simulink model "Force_control"  (R2020a)
settings: Solver=VariableStepAuto  StartTime=0.0  StopTime=10.0  RelTol=1e-3
values from neighbouring files (symbols this model uses):
  K = [C11 C12 C13 0 0 0; C12 C11 C13 0 0 0; C13 C13 C33 0 0 0; 0 0 0 C44 0 0; 0 0 0 0 C44 0; 0 0 0 0 0 C66]    [JoinScript.m]    (also in alldata.mat = [20.1 11.1 12 0 0 0 11.1 20.1 12 0 0 0 ... (36 elements, 6x6; aux_y2.m = Abb.fkine(q))
  Kd = 25*diag([1 1 1 1 1 1])    [JoinScript.m]    (also in alldata.mat = [150 0 0 0 0 0 0 150 0 0 0 0 ... (36 elements, 6x6)]; aux_y.m = 3e2*diag([1 1 1 1 1 1]); aux_y2.m = 3e2*diag([1 1 1 1 1 1]))
  Kp = 100*diag([0.01 1 1 1 1 1])    [JoinScript.m]    (also in alldata.mat = [200 0 0 0 0 0 0 200 0 0 0 0 ... (36 elements, 6x6)]; aux_y.m = 1e3*diag([1 1 1 1 1 1]); aux_y2.m = 1e3*diag([1 1 1 1 1 1]))
  x0 = dir_kin(qf)    [JoinScript.m]    (also in alldata.mat = [-5.32301496588e-18 0.480120382501 0.16494818601 1.570796326)
settings Model: Creator=doble  LastModifiedBy=doble

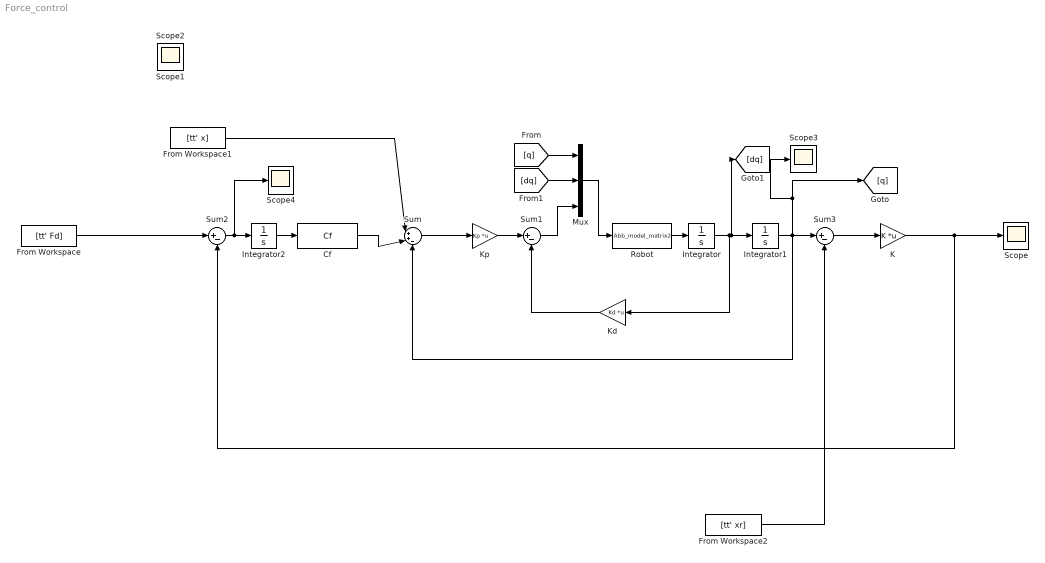
== system Force_control ==
  Cf : MATLABFcn  MATLABFcn=Cf  OutputDimensions=6*1
  From Workspace : FromWorkspace  VariableName=[tt' Fd]
  From Workspace1 : FromWorkspace  VariableName=[tt' x]
  From Workspace2 : FromWorkspace  VariableName=[tt' xr]
  Integrator : Integrator
  Integrator1 : Integrator  InitialCondition=x0
  Integrator2 : Integrator
  K : Gain  Gain=K  Multiplication=Matrix(K*u)
  Kd : Gain  Gain=Kd  Multiplication=Matrix(K*u)
  Kp : Gain  Gain=Kp  Multiplication=Matrix(K*u)
  Mux : Mux  Inputs=3
  Robot : MATLABFcn  MATLABFcn=Abb_model_matrix2  OutputDimensions=6*1
  Scope{,1..4} (5 alike) : Scope
  Sum : Sum  Inputs=|++-
  Sum1 : Sum  Inputs=|+-
  Sum2 : Sum  Inputs=|+-
  Sum3 : Sum  Inputs=|+-
  wires:
  From Workspace1/1 -> Sum/1
  Cf/1 -> Sum/2
  Sum/1 -> Kp/1
  Sum3/1 -> K/1
  Kp/1 -> Sum1/1
  Integrator/1 -> Kd/1, [dq], Integrator1/1
  Integrator1/1 -> [q], Scope3/1, Sum/3, Sum3/1
  Kd/1 -> Sum1/2
  K/1 -> Sum2/2, Scope/1
  From Workspace2/1 -> Sum3/2
  Integrator2/1 -> Cf/1
  Sum2/1 -> Scope4/1, Integrator2/1
  From Workspace/1 -> Sum2/1
  Robot/1 -> Integrator/1
  Mux/1 -> Robot/1
  Sum1/1 -> Mux/3
  [q] -> Mux/1
  [dq] -> Mux/2
